simulink model "massbalancer"  (R2024a)
settings: Solver=VariableStepAuto  StartTime=0.0  StopTime=inf  RelTol=1e-3
libraries: matrix_library x36, sharedutil x2, sharedtransform x2, dspinverses x1, aerolibutil x1
(part 1 of 3)
settings Model: Creator=robertbergbaum  LastModifiedBy=robertbergbaum

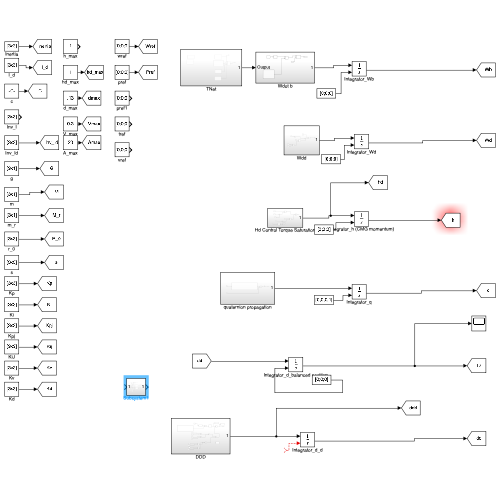
[thumbnail: Simulink's stored preview of the top-level diagram]
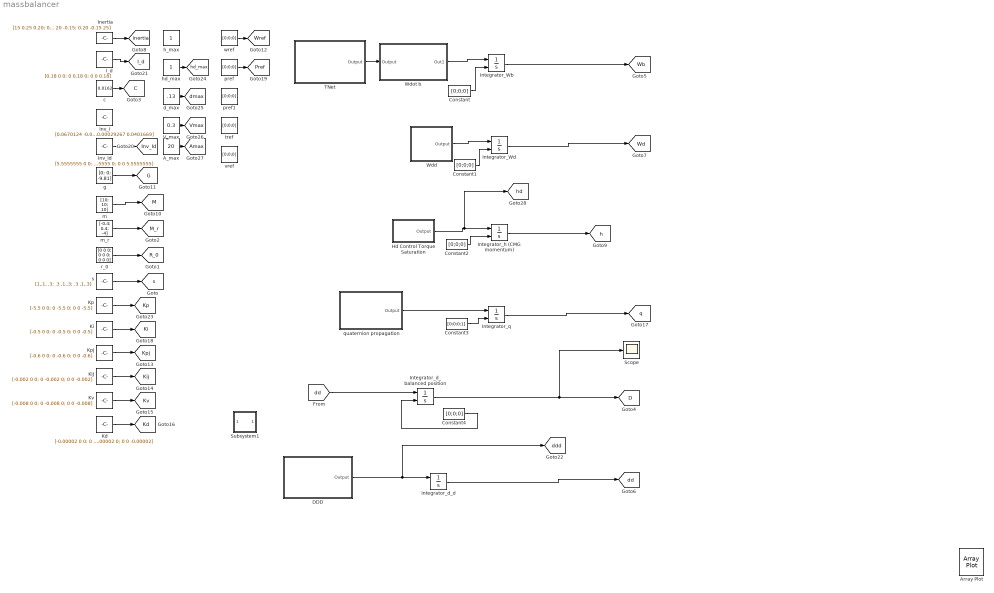
== system massbalancer ==
  A_max : Constant  Value=20
  Constant{,1..2,4} (4 alike) : Constant  Value=[0;0;0]  VectorParams1D=off
  Constant3 : Constant  Value=[0;0;0;1]  VectorParams1D=off
  DDD : Subsystem
  Hd Control Torque Saturation : Subsystem
  I_d : Constant  Value=[0.18 0 0; 0 0.18 0; 0 0 0.18]
  Inertia : Constant  Value=[15 0.25 0.20; 0.25 20 -0.15; 0.20 -0.15 25]  VectorParams1D=off
  Integrator_Wb : Integrator  InitialConditionSource=external  InitialCondition=[0;0;0]
  Integrator_Wd : Integrator  InitialConditionSource=external  InitialCondition=[0;0;0]
  Integrator_d_balanced position : Integrator  InitialConditionSource=external  InitialCondition=[0;0;0]
  Integrator_d_d : Integrator  InitialConditionSource=external  InitialCondition=[0;0;0]
  Integrator_h (CMG momentum) : Integrator  InitialConditionSource=external  InitialCondition=[0;0;0]
  Integrator_q : Integrator  InitialConditionSource=external  InitialCondition=[0;0;0;1]
  Inv_I : Constant  Value=[0.0670124 -0.0008106 -0.00051308; -0.0008106 0.0500357 0.00029267; -0.00051308 0.00029267 0.0401669]
  Inv_Id : Constant  Value=[5.5555555 0 0; 0 5.5555555 0; 0 0 5.5555555]
  Kd : Constant  Value=[-0.00002 0 0; 0 -0.00002 0; 0 0 -0.00002]
  Ki : Constant  Value=[-0.5 0 0; 0 -0.5 0; 0 0 -0.5]
  KiJ : Constant  Value=[-0.002 0 0; 0 -0.002 0; 0 0 -0.002]
  Kp : Constant  Value=[-5.5 0 0; 0 -5.5 0; 0 0 -5.5]
  Kpj : Constant  Value=[-0.6 0 0; 0 -0.6 0; 0 0 -0.6]
  Kv : Constant  Value=[-0.008 0 0; 0 -0.008 0; 0 0 -0.008]
  Scope : Scope
  Subsystem1 : Subsystem
  TNet : Subsystem
  V_max : Constant  Value=0.3
  Wdd : Subsystem
  Wdot b : Subsystem
  c : Constant  Value=0.0162  VectorParams1D=off
  d_max : Constant  Value=.13
  g : Constant  Value=[0; 0; -9.81]  VectorParams1D=off
  h_max : Constant
  hd_max : Constant
  m : Constant  Value=[10; 10; 10]  VectorParams1D=off
  m_r : Constant  Value=[-0.4; 0.4; -4]  VectorParams1D=off
  pref : Constant  Value=[0;0;0]  VectorParams1D=off
  pref1 : Constant  Value=[0;0;0]
  quaternion propagation : Subsystem
  r_0 : Constant  Value=[0 0 0; 0 0 0; 0 0 0]
  s : Constant  Value=[1,.1, .3; .3 ,1,.3; .3 ,1,.3]  VectorParams1D=off
  tref : Constant  Value=[0;0;0]
  vref : Constant  Value=[0;0;0]
  wref : Constant  Value=[0;0;0]  VectorParams1D=off
  Array Plot : ArrayPlot  IOType=viewer  IsFloating=on  WindowPosition=[447.000000,282.000000,800.000000,500.000000,]  ScopeFrameLocation=window  YLimits=[-4.3585 5.1367]  DefaultConfigurationName=dsp.scopes.ArrayPlotBlockSpecification
  tag scope: Amax=global, C=global, D=global, G=global, I_d=global, Inv_Id=global, Kd=global, Ki=global, Kij=global, Kp=global, Kpj=global, Kv=global, M=global, M_r=global, Pref=global, R_0=global, Vmax=global, Wb=global, Wd=global, Wref=global, dd=global, ddd=global, dmax=global, h=global, hd=global, hd_max=global, inertia=global, q=global, s=global
  wires:
  Integrator_Wb/1 -> [Wb]
  Kp/1 -> [Kp]
  Integrator_q/1 -> [q]
  Integrator_d_d/1 -> [dd]
  KiJ/1 -> [Kij]
  TNet/1(Output) -> Wdot b/1(Output)
  Ki/1 -> [Ki]
  s/1 -> [s]
  Constant2/1 -> Integrator_h (CMG momentum)/2
  r_0/1 -> [R_0]
  A_max/1 -> [Amax]
  Constant4/1 -> Integrator_d_balanced position/2
  I_d/1 -> [I_d]
  wref/1 -> [Wref]
  Inv_Id/1 -> [Inv_Id]
  [dd] -> Integrator_d_balanced position/1
  Wdot b/1(Out1) -> Integrator_Wb/1
  Integrator_d_balanced position/1 -> Scope/1, [D]
  DDD/1(Output) -> [ddd], Integrator_d_d/1
  Kd/1 -> [Kd]
  m/1 -> [M]
  pref/1 -> [Pref]
  Kpj/1 -> [Kpj]
  Kv/1 -> [Kv]
  Constant/1 -> Integrator_Wb/2
  Inertia/1 -> [inertia]
  c/1 -> [C]
  ? -> Integrator_d_d/2
  m_r/1 -> [M_r]
  Integrator_Wd/1 -> [Wd]
  Constant1/1 -> Integrator_Wd/2
  Wdd/1(Output) -> Integrator_Wd/1
  quaternion propagation/1(Output) -> Integrator_q/1
  g/1 -> [G]
  Hd Control Torque Saturation/1(Output) -> [hd], Integrator_h (CMG momentum)/1
  Integrator_h (CMG momentum)/1 -> [h]
  hd_max/1 -> [hd_max]
  Constant3/1 -> Integrator_q/2
  V_max/1 -> [Vmax]
  d_max/1 -> [dmax]

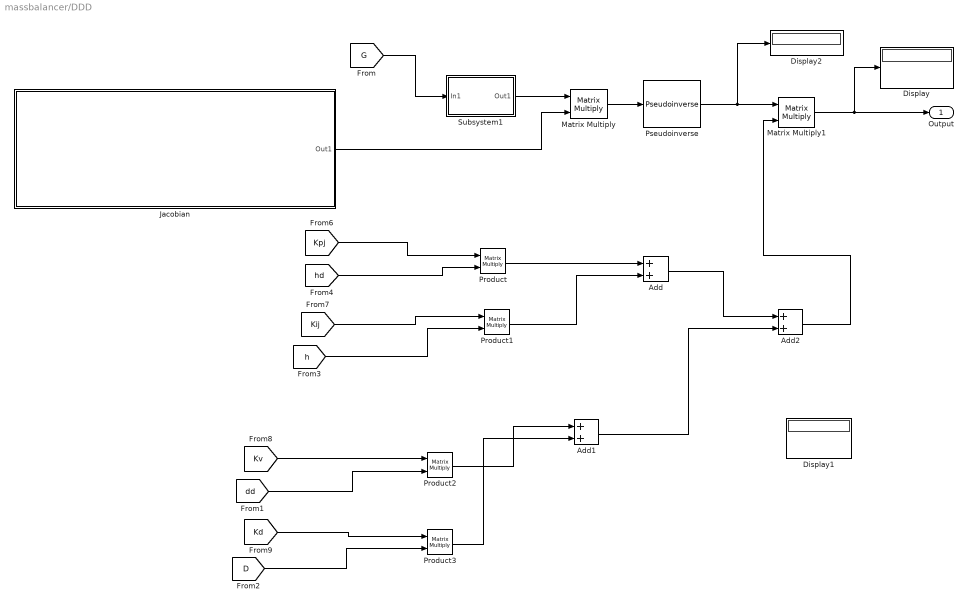
== system massbalancer/DDD ==
  Add : Sum
  Add1 : Sum
  Add2 : Sum
  Display : Display
  Display1 : Display
  Display2 : Display
  Jacobian : Subsystem
  Matrix Multiply : Product  Multiplication=Matrix(*)
  Matrix Multiply1 : Product  Multiplication=Matrix(*)
  Product{,1..3} (4 alike) : Product  Multiplication=Matrix(*)
  Pseudoinverse : dspinverses/Pseudoinverse  wanterr=off  SimulateUsing=Interpreted execution
  Subsystem1 : Subsystem
  Output : Outport
  wires:
  [Kij] -> Product1/1
  Add2/1 -> Matrix Multiply1/2
  Matrix Multiply/1 -> Pseudoinverse/1
  [Kpj] -> Product/1
  [h] -> Product1/2
  [G] -> Subsystem1/1(In1)
  [Kd] -> Product3/1
  [Kv] -> Product2/1
  [dd] -> Product2/2
  Subsystem1/1(Out1) -> Matrix Multiply/1
  Pseudoinverse/1 -> Display2/1, Matrix Multiply1/1
  Jacobian/1(Out1) -> Matrix Multiply/2
  Matrix Multiply1/1 -> Display/1, Output/1
  [D] -> Product3/2
  [hd] -> Product/2
  Product1/1 -> Add/2
  Product/1 -> Add/1
  Product2/1 -> Add1/1
  Product3/1 -> Add1/2
  Add/1 -> Add2/1
  Add1/1 -> Add2/2

== system massbalancer/Hd Control Torque Saturation ==
  Add : Sum
  Gain : Gain  Gain=2
  Matrix Multiply : Product  Multiplication=Matrix(*)
  Matrix Multiply1 : Product  Multiplication=Matrix(*)
  Selector : Selector  InputPortWidth=4  IndexOptions=Index vector (dialog)  Indices=[1 2 3]  OutputSizes=1
  Sum : Sum  Inputs=|+-
  Sum1 : Sum  Inputs=|+-
  Output : Outport
  wires:
  [q] -> Selector/1
  Selector/1 -> Gain/1
  Gain/1 -> Sum/2
  [Pref] -> Sum/1
  [Ki] -> Matrix Multiply/1
  Sum/1 -> Matrix Multiply/2
  [Wref] -> Sum1/1
  [Wb] -> Sum1/2
  [Kp] -> Matrix Multiply1/1
  Sum1/1 -> Matrix Multiply1/2
  Matrix Multiply1/1 -> Add/1
  Matrix Multiply/1 -> Add/2
  Add/1 -> Output/1

== system massbalancer/Subsystem1 ==
  In1 : Inport
  Demux : Demux  Outputs=3
  Demux1 : Demux  Outputs=3
  Demux4 : Demux  Outputs=3
  Mux : Mux  Inputs=3
  Subsystem1 : Subsystem
  Subsystem2 : Subsystem
  Subsystem3 : Subsystem
  Out1 : Outport
  wires:
  Demux/3 -> Subsystem3/6(ddd)
  Demux/2 -> Subsystem1/6(ddd)
  Demux/1 -> Subsystem2/5(ddd)
  Subsystem2/1(Out1) -> Mux/1
  Subsystem1/1(Out1) -> Mux/2
  Mux/1 -> Out1/1
  In1/1 -> Demux/1
  Subsystem3/1(Out1) -> Mux/3
  [D] -> Demux1/1
  Demux1/1 -> Subsystem2/1(d)
  [dd] -> Demux4/1
  Demux4/1 -> Subsystem2/3(dd)
  Demux1/2 -> Subsystem1/1(d)
  Demux4/2 -> Subsystem1/3(dd)
  [Amax] -> Subsystem2/6(amax), Subsystem1/5(amax), Subsystem3/5(amax)
  [Vmax] -> Subsystem3/4(vmax), Subsystem1/4(vmax), Subsystem2/4(vmax)
  Demux4/3 -> Subsystem3/3(dd)
  [dmax] -> Subsystem2/2(dmax), Subsystem3/2(dmax), Subsystem1/2(dmax)
  Demux1/3 -> Subsystem3/1(d)

== system massbalancer/TNet ==
  Add : Sum  Inputs=++--
  Hd Control Torque Saturation : Subsystem
  Subsystem : Subsystem
  Subsystem1 : Subsystem
  TBalances : Subsystem
  "Tbalances Init T Gravity " : Subsystem
  Tdamp : Subsystem
  Output : Outport
  tag scope: Tdamp=global
  wires:
  Tdamp/1(Outport) -> Add/1, [Tdamp]
  Subsystem/1(Out1) -> Add/3
  Hd Control Torque Saturation/1(Output) -> Add/4
  Add/1 -> Output/1
  Subsystem1/1(Output) -> Add/2

== system massbalancer/Wdd ==
  Cross Product : matrix_library/Cross Product
  Gain : Gain  Gain=-1
  Matrix Multiply : Product  Multiplication=Matrix(*)
  Matrix Multiply1 : Product  Multiplication=Matrix(*)
  Sum : Sum  Inputs=|+-
  Output : Outport
  wires:
  [Wb] -> Cross Product/1
  [Wd] -> Matrix Multiply/2
  [I_d] -> Matrix Multiply/1
  Matrix Multiply/1 -> Cross Product/2
  [Tdamp] -> Gain/1
  Gain/1 -> Sum/1
  Cross Product/1 -> Sum/2
  Sum/1 -> Matrix Multiply1/2
  [Inv_Id] -> Matrix Multiply1/1
  Matrix Multiply1/1 -> Output/1

== system massbalancer/Wdot b ==
  Output : Inport
  I_r : Subsystem
  Invert 3x3 Matrix : aerolibutil/Invert  3x3 Matrix
  Matrix Multiply : Product  Multiplication=Matrix(*)
  Subtract : Sum  Inputs=+-
  Out1 : Outport
  wires:
  Matrix Multiply/1 -> Out1/1
  I_r/1(Out1) -> Subtract/2
  Subtract/1 -> Matrix Multiply/1
  Output/1 -> Matrix Multiply/2
  [inertia] -> Invert 3x3 Matrix/1
  Invert 3x3 Matrix/1 -> Subtract/1

== system massbalancer/quaternion propagation ==
  Matrix Multiply : Product  Multiplication=Matrix(*)
  Multiply : Gain  Gain=0.5
  Omega Wb : Subsystem
  Output : Outport
  wires:
  [Wb] -> Omega Wb/1(In1)
  Multiply/1 -> Output/1
  Omega Wb/1(Output) -> Matrix Multiply/1
  Matrix Multiply/1 -> Multiply/1
  [q] -> Matrix Multiply/2

== system massbalancer/DDD/Jacobian ==
  Gain : Gain  Gain=-1
  Matrix Concatenate : Concatenate  NumInputs=3  Mode=Multidimensional array  ConcatenateDimension=2
  Product : Product
  Product1 : Product
  Product2 : Product
  Selector : Selector  InputPortWidth=3  IndexOptions=Index vector (dialog)  Indices=[1]  OutputSizes=1
  Selector1 : Selector  InputPortWidth=3  IndexOptions=Index vector (dialog)  Indices=[2]  OutputSizes=1
  Selector2 : Selector  InputPortWidth=3  IndexOptions=Index vector (dialog)  Indices=[3]  OutputSizes=1
  Subsystem1 : Subsystem
  Out1 : Outport
  wires:
  Product1/1 -> Matrix Concatenate/2
  Subsystem1/2(Out2) -> Product1/1
  Subsystem1/1(Out1) -> Product/1
  Product2/1 -> Matrix Concatenate/3
  Selector2/1 -> Product2/2
  Selector/1 -> Product/2
  Matrix Concatenate/1 -> Gain/1
  Selector1/1 -> Product1/2
  [M] -> Selector/1, Selector2/1, Selector1/1
  Gain/1 -> Out1/1
  Product/1 -> Matrix Concatenate/1
  Subsystem1/3(Out3) -> Product2/1
  [s] -> Subsystem1/1(R_0)

== system massbalancer/DDD/Subsystem1 ==
  In1 : Inport
  Constant : Constant  Value=0  VectorParams1D=off
  Constant1 : Constant  Value=0  VectorParams1D=off
  Constant2 : Constant  Value=0  VectorParams1D=off
  Demux : Demux  Outputs=3
  Gain : Gain  Gain=-1
  Gain1 : Gain  Gain=-1
  Gain2 : Gain  Gain=-1
  Matrix Concatenate : Concatenate  NumInputs=3  Mode=Multidimensional array  ConcatenateDimension=2
  Mux : Mux  Inputs=3
  Mux1 : Mux  Inputs=3
  Mux2 : Mux  Inputs=3
  Out1 : Outport
  wires:
  Matrix Concatenate/1 -> Out1/1
  Constant2/1 -> Mux2/3
  Constant1/1 -> Mux1/2
  Demux/1 -> Gain1/1, Mux2/2
  Mux2/1 -> Matrix Concatenate/3
  Demux/3 -> Gain/1, Mux1/1
  Gain/1 -> Mux/2
  In1/1 -> Demux/1
  Demux/2 -> Gain2/1, Mux/3
  Mux/1 -> Matrix Concatenate/1
  Gain1/1 -> Mux1/3
  Gain2/1 -> Mux2/1
  Constant/1 -> Mux/1
  Mux1/1 -> Matrix Concatenate/2

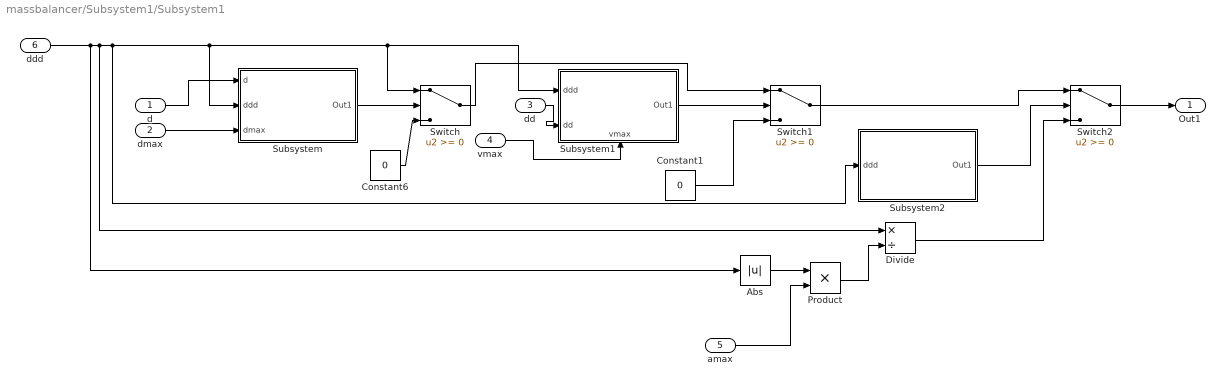
== system massbalancer/Subsystem1/Subsystem1 ==
  d : Inport
  dmax : Inport  Port=2
  dd : Inport  Port=3
  vmax : Inport  Port=4
  amax : Inport  Port=5
  ddd : Inport  Port=6
  Abs : Abs  SaturateOnIntegerOverflow=off
  Constant1 : Constant  Value=0  VectorParams1D=off
  Constant6 : Constant  Value=0  VectorParams1D=off
  Divide : Product  Inputs=*/
  Product : Product
  Subsystem : Subsystem
  Subsystem1 : Subsystem
      settings: PortSchema="{\"entries\":[{\"content\":{\"sides\":[{\"content\":{\"connectorIds\":[\"In1\",\"In2\"]},\"type\":\"ConnectorPlacement.EquallySpacedRectSide\",\"uuid\":\"8ae5d5fe-f648-4880-a31b-82c697ea1f6b\"},{\"content\":{\"connectorIds\":[\"Out1\"],\"side\":\"RIGHT\"},\"type\":\"ConnectorPlacement.EquallySpacedRectSide\",\"uuid\":\"93459a1a-512a-419a-be8d-aafe7ca608a5\"},{\"content\":{\"side\":\"TOP\"},\"type\":\"ConnectorPlacement.EquallySpacedRectSide\",\"uuid\":\"819310a9-1bbe-4933-988e-a24734f33f30\"},{\"content\":{\"connectorIds\":[\"In3\"],\"side\":\"BOTTOM\"},\"type\":\"ConnectorPlacement.EquallySpacedRectSide\",\"uuid\":\"b19b6ff1-25c5-41e7-8899-8dec42881787\"}]},\"type\":\"ConnectorPlacement.EquallySpacedConnector\",\"uuid\":\"36ccd371-697e-4cae-b4c0-046b64d9372c\"}],\"packageUris\":[\"http://schema.mathworks.com/mf0/Connector/R2020b\"],\"version\":\"1.0\"}"
  Subsystem2 : Subsystem
  Switch : Switch  SaturateOnIntegerOverflow=off  InputSameDT=off
  Switch1 : Switch  SaturateOnIntegerOverflow=off  InputSameDT=off
  Switch2 : Switch  SaturateOnIntegerOverflow=off  InputSameDT=off
  Out1 : Outport
  wires:
  vmax/1 -> Subsystem1/3(vmax)
  dd/1 -> Subsystem1/2(dd)
  dmax/1 -> Subsystem/3(dmax)
  d/1 -> Subsystem/1(d)
  Switch1/1 -> Switch2/1
  Switch/1 -> Switch1/1
  Constant6/1 -> Switch/3
  Product/1 -> Divide/2
  Switch2/1 -> Out1/1
  Divide/1 -> Switch2/3
  ddd/1 -> Switch/1, Subsystem1/1(ddd), Subsystem/2(ddd), Subsystem2/1(ddd), Divide/1, Abs/1
  Subsystem/1(Out1) -> Switch/2
  Subsystem2/1(Out1) -> Switch2/2
  amax/1 -> Product/2
  Subsystem1/1(Out1) -> Switch1/2
  Constant1/1 -> Switch1/3
  Abs/1 -> Product/1

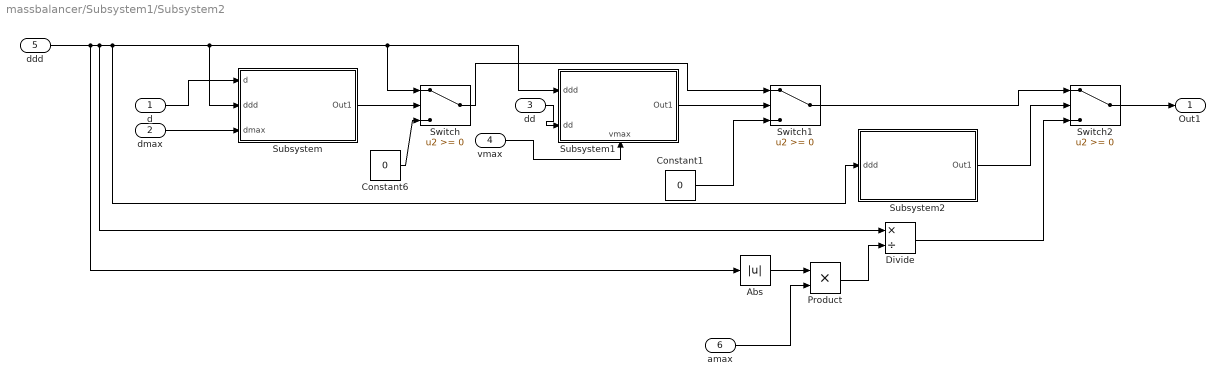
== system massbalancer/Subsystem1/Subsystem2 ==
  d : Inport
  dmax : Inport  Port=2
  dd : Inport  Port=3
  vmax : Inport  Port=4
  ddd : Inport  Port=5
  amax : Inport  Port=6
  Abs : Abs  SaturateOnIntegerOverflow=off
  Constant1 : Constant  Value=0  VectorParams1D=off
  Constant6 : Constant  Value=0  VectorParams1D=off
  Divide : Product  Inputs=*/
  Product : Product
  Subsystem : Subsystem
  Subsystem1 : Subsystem
      settings: PortSchema="{\"entries\":[{\"content\":{\"sides\":[{\"content\":{\"connectorIds\":[\"In1\",\"In2\"]},\"type\":\"ConnectorPlacement.EquallySpacedRectSide\",\"uuid\":\"8ae5d5fe-f648-4880-a31b-82c697ea1f6b\"},{\"content\":{\"connectorIds\":[\"Out1\"],\"side\":\"RIGHT\"},\"type\":\"ConnectorPlacement.EquallySpacedRectSide\",\"uuid\":\"93459a1a-512a-419a-be8d-aafe7ca608a5\"},{\"content\":{\"side\":\"TOP\"},\"type\":\"ConnectorPlacement.EquallySpacedRectSide\",\"uuid\":\"819310a9-1bbe-4933-988e-a24734f33f30\"},{\"content\":{\"connectorIds\":[\"In3\"],\"side\":\"BOTTOM\"},\"type\":\"ConnectorPlacement.EquallySpacedRectSide\",\"uuid\":\"b19b6ff1-25c5-41e7-8899-8dec42881787\"}]},\"type\":\"ConnectorPlacement.EquallySpacedConnector\",\"uuid\":\"36ccd371-697e-4cae-b4c0-046b64d9372c\"}],\"packageUris\":[\"http://schema.mathworks.com/mf0/Connector/R2020b\"],\"version\":\"1.0\"}"
  Subsystem2 : Subsystem
  Switch : Switch  SaturateOnIntegerOverflow=off  InputSameDT=off
  Switch1 : Switch  SaturateOnIntegerOverflow=off  InputSameDT=off
  Switch2 : Switch  SaturateOnIntegerOverflow=off  InputSameDT=off
  Out1 : Outport
  wires:
  Abs/1 -> Product/1
  Constant1/1 -> Switch1/3
  Subsystem1/1(Out1) -> Switch1/2
  amax/1 -> Product/2
  Subsystem2/1(Out1) -> Switch2/2
  Subsystem/1(Out1) -> Switch/2
  ddd/1 -> Abs/1, Divide/1, Subsystem2/1(ddd), Subsystem/2(ddd), Subsystem1/1(ddd), Switch/1
  Divide/1 -> Switch2/3
  Switch2/1 -> Out1/1
  Product/1 -> Divide/2
  Constant6/1 -> Switch/3
  Switch/1 -> Switch1/1
  Switch1/1 -> Switch2/1
  d/1 -> Subsystem/1(d)
  dmax/1 -> Subsystem/3(dmax)
  dd/1 -> Subsystem1/2(dd)
  vmax/1 -> Subsystem1/3(vmax)

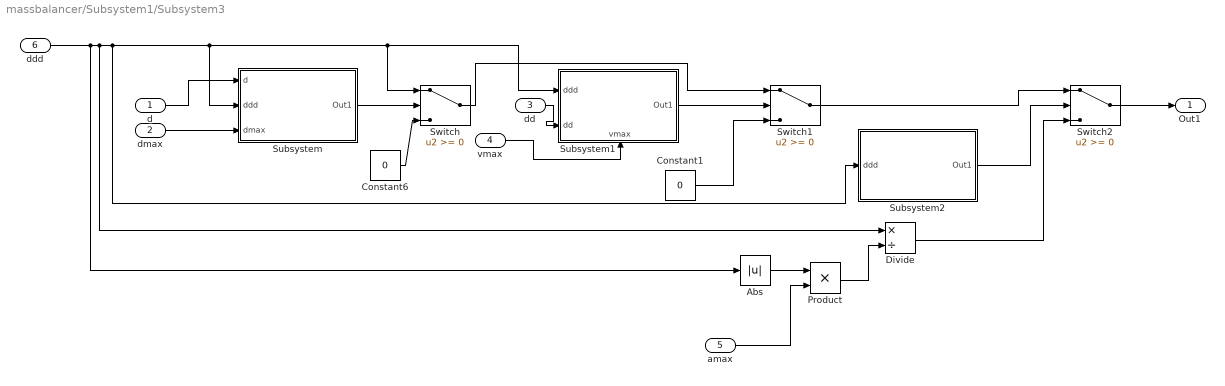
== system massbalancer/Subsystem1/Subsystem3 ==
  d : Inport
  dmax : Inport  Port=2
  dd : Inport  Port=3
  vmax : Inport  Port=4
  amax : Inport  Port=5
  ddd : Inport  Port=6
  Abs : Abs  SaturateOnIntegerOverflow=off
  Constant1 : Constant  Value=0  VectorParams1D=off
  Constant6 : Constant  Value=0  VectorParams1D=off
  Divide : Product  Inputs=*/
  Product : Product
  Subsystem : Subsystem
  Subsystem1 : Subsystem
      settings: PortSchema="{\"entries\":[{\"content\":{\"sides\":[{\"content\":{\"connectorIds\":[\"In1\",\"In2\"]},\"type\":\"ConnectorPlacement.EquallySpacedRectSide\",\"uuid\":\"8ae5d5fe-f648-4880-a31b-82c697ea1f6b\"},{\"content\":{\"connectorIds\":[\"Out1\"],\"side\":\"RIGHT\"},\"type\":\"ConnectorPlacement.EquallySpacedRectSide\",\"uuid\":\"93459a1a-512a-419a-be8d-aafe7ca608a5\"},{\"content\":{\"side\":\"TOP\"},\"type\":\"ConnectorPlacement.EquallySpacedRectSide\",\"uuid\":\"819310a9-1bbe-4933-988e-a24734f33f30\"},{\"content\":{\"connectorIds\":[\"In3\"],\"side\":\"BOTTOM\"},\"type\":\"ConnectorPlacement.EquallySpacedRectSide\",\"uuid\":\"b19b6ff1-25c5-41e7-8899-8dec42881787\"}]},\"type\":\"ConnectorPlacement.EquallySpacedConnector\",\"uuid\":\"36ccd371-697e-4cae-b4c0-046b64d9372c\"}],\"packageUris\":[\"http://schema.mathworks.com/mf0/Connector/R2020b\"],\"version\":\"1.0\"}"
  Subsystem2 : Subsystem
  Switch : Switch  SaturateOnIntegerOverflow=off  InputSameDT=off
  Switch1 : Switch  SaturateOnIntegerOverflow=off  InputSameDT=off
  Switch2 : Switch  SaturateOnIntegerOverflow=off  InputSameDT=off
  Out1 : Outport
  wires:
  Abs/1 -> Product/1
  Constant1/1 -> Switch1/3
  Subsystem1/1(Out1) -> Switch1/2
  amax/1 -> Product/2
  Subsystem2/1(Out1) -> Switch2/2
  Subsystem/1(Out1) -> Switch/2
  ddd/1 -> Abs/1, Divide/1, Subsystem2/1(ddd), Subsystem/2(ddd), Subsystem1/1(ddd), Switch/1
  Divide/1 -> Switch2/3
  Switch2/1 -> Out1/1
  Product/1 -> Divide/2
  Constant6/1 -> Switch/3
  Switch/1 -> Switch1/1
  Switch1/1 -> Switch2/1
  d/1 -> Subsystem/1(d)
  dmax/1 -> Subsystem/3(dmax)
  dd/1 -> Subsystem1/2(dd)
  vmax/1 -> Subsystem1/3(vmax)

== system massbalancer/TNet/Hd Control Torque Saturation ==
  Add : Sum
  Gain : Gain  Gain=2
  Matrix Multiply : Product  Multiplication=Matrix(*)
  Matrix Multiply1 : Product  Multiplication=Matrix(*)
  Selector : Selector  InputPortWidth=4  IndexOptions=Index vector (dialog)  Indices=[1 2 3]  OutputSizes=1
  Sum : Sum  Inputs=|+-
  Sum1 : Sum  Inputs=|+-
  Output : Outport
  wires:
  [q] -> Selector/1
  Selector/1 -> Gain/1
  Gain/1 -> Sum/2
  [Pref] -> Sum/1
  [Ki] -> Matrix Multiply/1
  Sum/1 -> Matrix Multiply/2
  [Wref] -> Sum1/1
  [Wb] -> Sum1/2
  [Kp] -> Matrix Multiply1/1
  Sum1/1 -> Matrix Multiply1/2
  Matrix Multiply1/1 -> Add/1
  Matrix Multiply/1 -> Add/2
  Add/1 -> Output/1

== system massbalancer/TNet/Subsystem ==
  Cross Product : matrix_library/Cross Product
  Product : Product  Multiplication=Matrix(*)
  Sum : Sum  Inputs=|++
  Out1 : Outport
  wires:
  Product/1 -> Sum/1
  [h] -> Sum/2
  Cross Product/1 -> Out1/1
  [inertia] -> Product/1
  Sum/1 -> Cross Product/2
  [Wb] -> Cross Product/1
  [Wb] -> Product/2

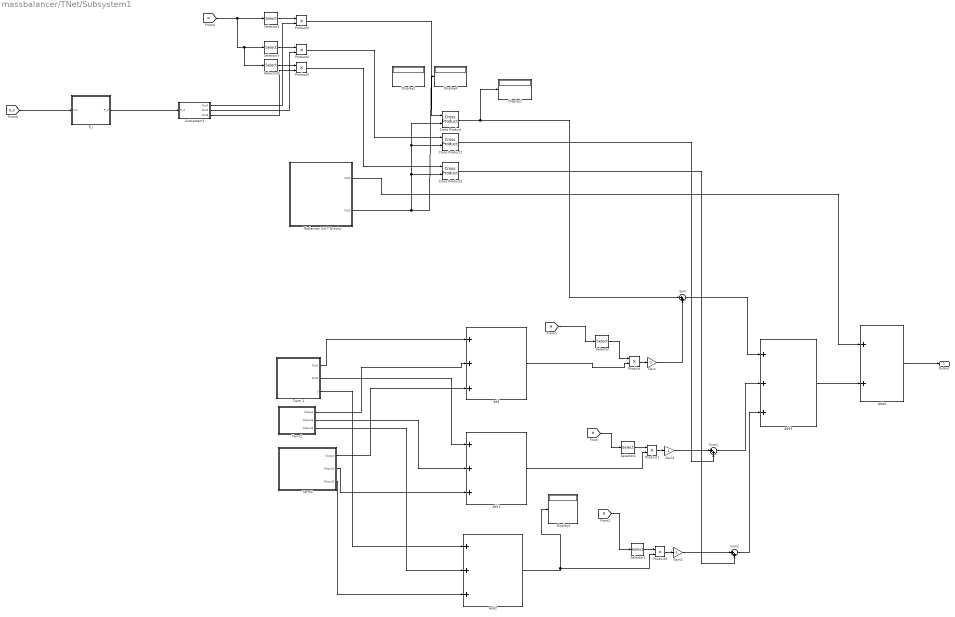
== system massbalancer/TNet/Subsystem1 ==
  Add{,1..3} (4 alike) : Sum  Inputs=+++
  Add4 : Sum
  Cross Product : matrix_library/Cross Product
  Cross Product1 : matrix_library/Cross Product
  Cross Product2 : matrix_library/Cross Product
  Display{1..4} (4 alike) : Display
  Gain : Gain  Gain=-1
  Gain1 : Gain  Gain=-1
  Gain2 : Gain  Gain=-1
  Product{,1..5} (6 alike) : Product
  R_I : Subsystem
  Selector : Selector  InputPortWidth=3  IndexOptions=Index vector (dialog)  Indices=[1]  OutputSizes=1
  Selector1 : Selector  InputPortWidth=3  IndexOptions=Index vector (dialog)  Indices=[2]  OutputSizes=1
  Selector2 : Selector  InputPortWidth=3  IndexOptions=Index vector (dialog)  Indices=[3]  OutputSizes=1
  Selector3 : Selector  InputPortWidth=3  IndexOptions=Index vector (dialog)  Indices=[2]  OutputSizes=1
  Selector4 : Selector  InputPortWidth=3  IndexOptions=Index vector (dialog)  Indices=[1]  OutputSizes=1
  Selector5 : Selector  InputPortWidth=3  IndexOptions=Index vector (dialog)  Indices=[3]  OutputSizes=1
  Subsystem3 : Subsystem
  Sum : Sum  Inputs=|++
  Sum1 : Sum  Inputs=|++
  Sum2 : Sum  Inputs=|++
  "Tbalances Init T Gravity " : Subsystem
  Term 1 : Subsystem
  Term2 : Subsystem
  Term3 : Subsystem
  Output : Outport
  wires:
  [M] -> Selector2/1
  Product2/1 -> Gain2/1
  Term 1/3(y) -> Add2/1
  Add1/1 -> Product1/2
  Sum1/1 -> Add3/2
  Add3/1 -> Add4/2
  Subsystem3/2(Out2) -> Product4/2
  Sum2/1 -> Add3/3
  "Tbalances Init T Gravity "/1(Out1) -> Add4/1
  Term3/2(Output1) -> Add1/3
  Subsystem3/3(Out3) -> Product5/2
  Cross Product/1 -> Display1/1, Sum/1
  Product4/1 -> Cross Product1/1
  Add4/1 -> Output/1
  Gain1/1 -> Sum1/1
  Cross Product2/1 -> Sum2/2
  [M] -> Selector1/1
  R_I/1(R_0) -> Subsystem3/1(R_0)
  Term2/1(Output) -> Add/2
  Term2/3(Output2) -> Add2/2
  Product5/1 -> Cross Product2/1
  Cross Product1/1 -> Sum1/2
  [M] -> Selector5/1, Selector3/1, Selector4/1
  Selector2/1 -> Product2/1
  Term2/2(Output1) -> Add1/2
  Term 1/1(Out1) -> Add/1
  Term3/1(Output) -> Add/3
  [R_0] -> R_I/1(In1)
  Selector4/1 -> Product3/1
  [M] -> Selector/1
  Product/1 -> Gain/1
  Term3/3(Output2) -> Add2/3
  "Tbalances Init T Gravity "/2(Out2) -> Display4/1, Cross Product2/2, Cross Product1/2, Cross Product/2
  Subsystem3/1(Out1) -> Product3/2
  Gain2/1 -> Sum2/1
  Selector/1 -> Product/1
  Add/1 -> Product/2
  Add2/1 -> Product2/2, Display3/1
  Term 1/2(Out2) -> Add1/1
  Selector3/1 -> Product4/1
  Product1/1 -> Gain1/1
  Product3/1 -> Cross Product/1
  Selector1/1 -> Product1/1
  Gain/1 -> Sum/2
  Selector5/1 -> Product5/1
  Sum/1 -> Add3/1

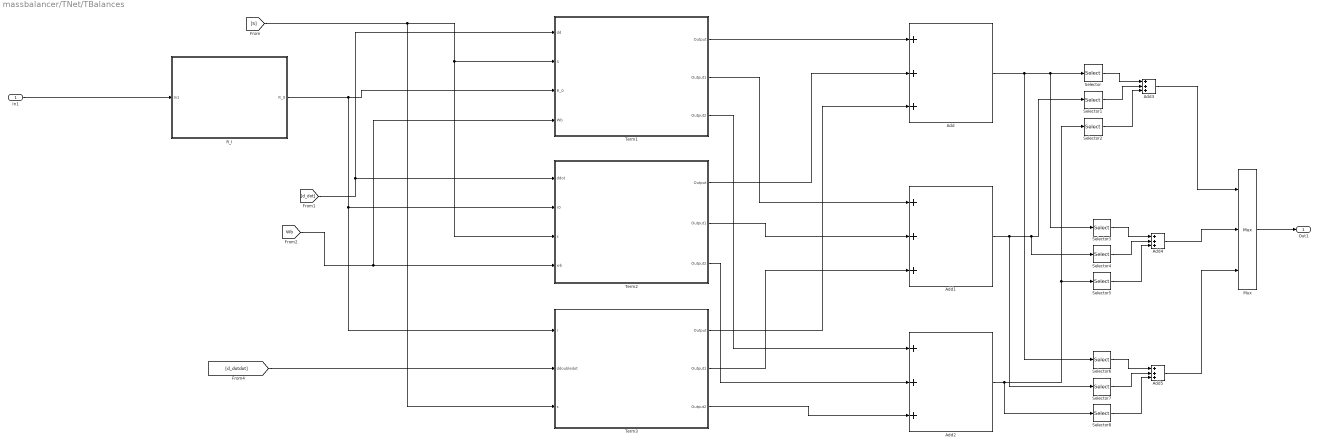
== system massbalancer/TNet/TBalances ==
  In1 : Inport
  Add{,1..5} (6 alike) : Sum  Inputs=+++
  Mux : Mux  Inputs=3
  R_I : Subsystem
  Selector : Selector  InputPortWidth=3  IndexOptions=Index vector (dialog)  Indices=[1 ]  OutputSizes=1
  Selector1 : Selector  InputPortWidth=3  IndexOptions=Index vector (dialog)  Indices=[1 ]  OutputSizes=1
  Selector2 : Selector  InputPortWidth=3  IndexOptions=Index vector (dialog)  Indices=[1 ]  OutputSizes=1
  Selector3 : Selector  InputPortWidth=3  IndexOptions=Index vector (dialog)  Indices=[2 ]  OutputSizes=1
  Selector4 : Selector  InputPortWidth=3  IndexOptions=Index vector (dialog)  Indices=[2]  OutputSizes=1
  Selector5 : Selector  InputPortWidth=3  IndexOptions=Index vector (dialog)  Indices=[2 ]  OutputSizes=1
  Selector6 : Selector  InputPortWidth=3  IndexOptions=Index vector (dialog)  Indices=[3 ]  OutputSizes=1
  Selector7 : Selector  InputPortWidth=3  IndexOptions=Index vector (dialog)  Indices=[3]  OutputSizes=1
  Selector8 : Selector  InputPortWidth=3  IndexOptions=Index vector (dialog)  Indices=[3 ]  OutputSizes=1
  Term1 : Subsystem
  Term2 : Subsystem
  Term3 : Subsystem
  Out1 : Outport
  wires:
  Add2/1 -> Selector8/1, Selector5/1, Selector2/1
  [d_dotdot] -> Term3/2(ddoubledot)
  Term1/3(Output2) -> Add2/1
  Add3/1 -> Mux/1
  Add4/1 -> Mux/2
  Selector7/1 -> Add5/2
  Term3/2(Output1) -> Add1/3
  [d_dot] -> Term2/1(ddot), Term1/1(dd)
  Term1/1(Output) -> Add/1
  Term2/1(Output) -> Add/2
  [S] -> Term3/3(s), Term2/3(s), Term1/2(S)
  Selector2/1 -> Add3/3
  Selector8/1 -> Add5/3
  Term3/1(Output) -> Add/3
  Selector/1 -> Add3/1
  Term2/2(Output1) -> Add1/2
  Add/1 -> Selector6/1, Selector3/1, Selector/1
  Selector3/1 -> Add4/1
  Add1/1 -> Selector7/1, Selector4/1, Selector1/1
  Selector1/1 -> Add3/2
  Selector4/1 -> Add4/2
  Selector6/1 -> Add5/1
  Term1/2(Output1) -> Add1/1
  Term3/3(Output2) -> Add2/3
  R_I/1(R_0) -> Term3/1(r), Term2/2(r0), Term1/3(R_0)
  [Wb] -> Term1/4(Wb), Term2/4(wb)
  Selector5/1 -> Add4/3
  Term2/3(Output2) -> Add2/2
  Add5/1 -> Mux/3
  In1/1 -> R_I/1(In1)
  Mux/1 -> Out1/1

== system massbalancer/TNet/Tbalances Init T Gravity  ==
  Fgravity : Subsystem
  Matrix Multiply : Product  Multiplication=Matrix(*)
  Subsystem : Subsystem
  Out1 : Outport
  wires:
  Subsystem/1(Output) -> Matrix Multiply/1
  Fgravity/1(Out1) -> Matrix Multiply/2
  Matrix Multiply/1 -> Out1/1

== system massbalancer/TNet/Tdamp ==
  Product : Product
  Subtract : Sum  Inputs=+-
  Outport : Outport
  wires:
  [Wb] -> Subtract/2
  [Wd] -> Subtract/1
  Subtract/1 -> Product/1
  [C] -> Product/2
  Product/1 -> Outport/1

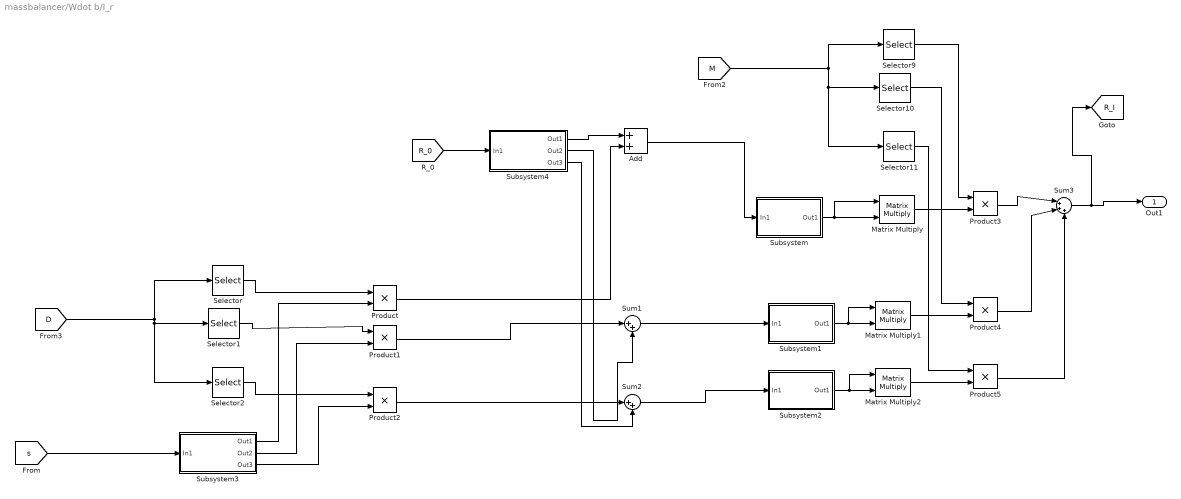
== system massbalancer/Wdot b/I_r ==
  Add : Sum
  Matrix Multiply : Product  Multiplication=Matrix(*)
  Matrix Multiply1 : Product  Multiplication=Matrix(*)
  Matrix Multiply2 : Product  Multiplication=Matrix(*)
  Product{,1..5} (6 alike) : Product
  Selector : Selector  InputPortWidth=3  IndexOptions=Index vector (dialog)  Indices=[1]  OutputSizes=1
  Selector1 : Selector  InputPortWidth=3  IndexOptions=Index vector (dialog)  Indices=[2]  OutputSizes=1
  Selector10 : Selector  InputPortWidth=3  IndexOptions=Index vector (dialog)  Indices=[2]  OutputSizes=1
  Selector11 : Selector  InputPortWidth=3  IndexOptions=Index vector (dialog)  Indices=[3]  OutputSizes=1
  Selector2 : Selector  InputPortWidth=3  IndexOptions=Index vector (dialog)  Indices=[3]  OutputSizes=1
  Selector9 : Selector  InputPortWidth=3  IndexOptions=Index vector (dialog)  Indices=[1]  OutputSizes=1
  Subsystem : Subsystem
  Subsystem1 : Subsystem
  Subsystem2 : Subsystem
  Subsystem3 : Subsystem
  Subsystem4 : Subsystem
  Sum1 : Sum  Inputs=|++
  Sum2 : Sum  Inputs=|++
  Sum3 : Sum  Inputs=|+++
  Out1 : Outport
  tag scope: R_I=global
  wires:
  Selector11/1 -> Product5/1
  Selector10/1 -> Product4/1
  Subsystem4/1(Out1) -> Add/1
  Subsystem/1(Out1) -> Matrix Multiply/1, Matrix Multiply/2
  Selector9/1 -> Product3/1
  Sum2/1 -> Subsystem2/1(In1)
  Matrix Multiply/1 -> Product3/2
  Matrix Multiply1/1 -> Product4/2
  Sum1/1 -> Subsystem1/1(In1)
  Product1/1 -> Sum1/1
  [M] -> Selector9/1, Selector11/1, Selector10/1
  Selector1/1 -> Product1/1
  Matrix Multiply2/1 -> Product5/2
  Add/1 -> Subsystem/1(In1)
  Selector/1 -> Product/1
  Product4/1 -> Sum3/2
  Subsystem3/2(Out2) -> Product1/2
  Product3/1 -> Sum3/1
  Selector2/1 -> Product2/1
  Subsystem4/2(Out2) -> Sum1/2
  [D] -> Selector/1, Selector1/1, Selector2/1
  Sum3/1 -> [R_I], Out1/1
  Product5/1 -> Sum3/3
  Subsystem4/3(Out3) -> Sum2/2
  Product/1 -> Add/2
  Subsystem3/1(Out1) -> Product/2
  [s] -> Subsystem3/1(In1)
  Subsystem3/3(Out3) -> Product2/2
  Subsystem2/1(Out1) -> Matrix Multiply2/1, Matrix Multiply2/2
  Product2/1 -> Sum2/1
  Subsystem1/1(Out1) -> Matrix Multiply1/1, Matrix Multiply1/2
  [R_0] -> Subsystem4/1(In1)

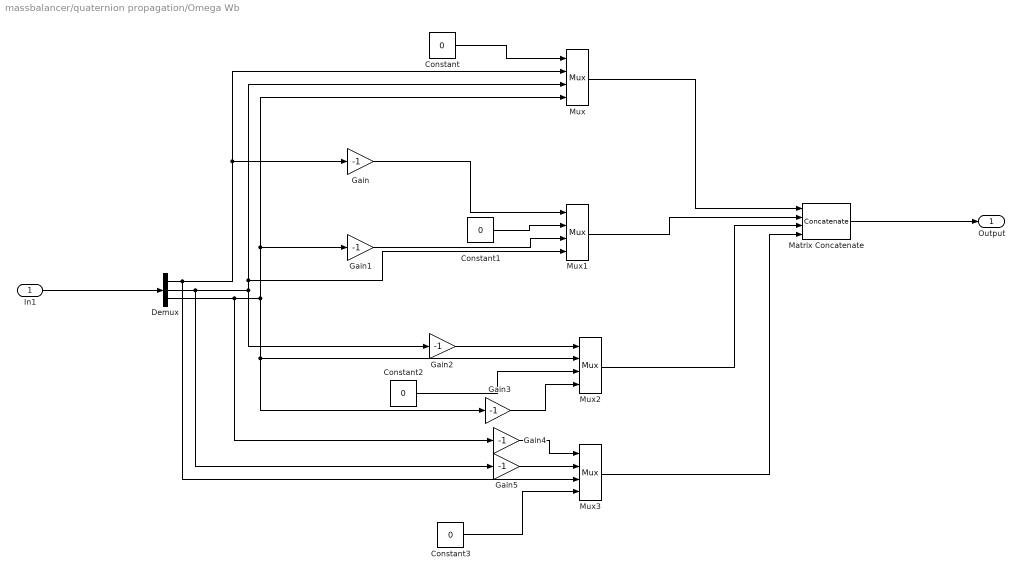
== system massbalancer/quaternion propagation/Omega Wb ==
  In1 : Inport
  Constant{,1..3} (4 alike) : Constant  Value=0  VectorParams1D=off
  Demux : Demux  Outputs=3
  Gain{,1..5} (6 alike) : Gain  Gain=-1
  Matrix Concatenate : Concatenate  NumInputs=4  Mode=Multidimensional array  ConcatenateDimension=2
  Mux{,1..3} (4 alike) : Mux
  Output : Outport
  wires:
  Constant/1 -> Mux/1
  In1/1 -> Demux/1
  Constant1/1 -> Mux1/2
  Gain1/1 -> Mux1/3
  Gain5/1 -> Mux3/2
  Gain/1 -> Mux1/1
  Mux2/1 -> Matrix Concatenate/3
  Demux/3 -> Gain4/1, Gain3/1, Mux2/2, Gain1/1, Mux/4
  Constant3/1 -> Mux3/4
  Constant2/1 -> Mux2/3
  Gain2/1 -> Mux2/1
  Mux3/1 -> Matrix Concatenate/4
  Gain4/1 -> Mux3/1
  Mux1/1 -> Matrix Concatenate/2
  Demux/1 -> Mux3/3, Gain/1, Mux/2
  Demux/2 -> Gain5/1, Mux/3, Mux1/4, Gain2/1
  Mux/1 -> Matrix Concatenate/1
  Gain3/1 -> Mux2/4
  Matrix Concatenate/1 -> Output/1

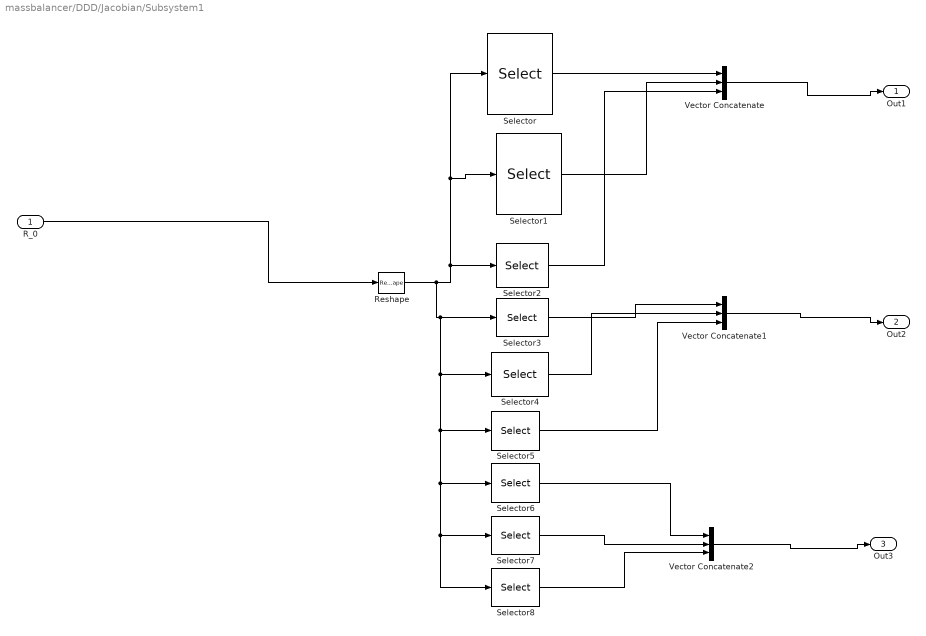
== system massbalancer/DDD/Jacobian/Subsystem1 ==
  R_0 : Inport
  Reshape : Reshape  OutputDimensionality=Column vector (2-D)  OutputDimensions=[1,3]
  Selector : Selector  InputPortWidth=9  IndexOptions=Index vector (dialog)  Indices=[1]  OutputSizes=1
  Selector1 : Selector  InputPortWidth=9  IndexOptions=Index vector (dialog)  Indices=[2]  OutputSizes=1
  Selector2 : Selector  InputPortWidth=9  IndexOptions=Index vector (dialog)  Indices=[3]  OutputSizes=1
  Selector3 : Selector  InputPortWidth=9  IndexOptions=Index vector (dialog)  Indices=[4]  OutputSizes=1
  Selector4 : Selector  InputPortWidth=9  IndexOptions=Index vector (dialog)  Indices=[5]  OutputSizes=1
  Selector5 : Selector  InputPortWidth=9  IndexOptions=Index vector (dialog)  Indices=[6]  OutputSizes=1
  Selector6 : Selector  InputPortWidth=9  IndexOptions=Index vector (dialog)  Indices=[7]  OutputSizes=1
  Selector7 : Selector  InputPortWidth=9  IndexOptions=Index vector (dialog)  Indices=[8]  OutputSizes=1
  Selector8 : Selector  InputPortWidth=9  IndexOptions=Index vector (dialog)  Indices=[9]  OutputSizes=1
  Vector Concatenate : Concatenate  NumInputs=3  Mode=Multidimensional array
  Vector Concatenate1 : Concatenate  NumInputs=3  Mode=Multidimensional array
  Vector Concatenate2 : Concatenate  NumInputs=3  Mode=Multidimensional array
  Out1 : Outport
  Out2 : Outport  Port=2
  Out3 : Outport  Port=3
  wires:
  Selector3/1 -> Vector Concatenate1/1
  Selector1/1 -> Vector Concatenate/2
  Vector Concatenate1/1 -> Out2/1
  Vector Concatenate2/1 -> Out3/1
  Selector7/1 -> Vector Concatenate2/2
  Selector5/1 -> Vector Concatenate1/3
  Selector/1 -> Vector Concatenate/1
  Reshape/1 -> Selector/1, Selector1/1, Selector2/1, Selector3/1, Selector4/1, Selector5/1, Selector6/1, Selector7/1, Selector8/1
  R_0/1 -> Reshape/1
  Selector6/1 -> Vector Concatenate2/1
  Selector4/1 -> Vector Concatenate1/2
  Selector8/1 -> Vector Concatenate2/3
  Vector Concatenate/1 -> Out1/1
  Selector2/1 -> Vector Concatenate/3

== system massbalancer/Subsystem1/Subsystem1/Subsystem ==
  d : Inport
  ddd : Inport  Port=2
  dmax : Inport  Port=3
  AND : Logic  IconShape=distinctive  AllPortsSameDT=off  OutDataTypeStr=boolean
  Abs : Abs  SaturateOnIntegerOverflow=off
  Constant : Constant  Value=0  VectorParams1D=off
  Constant1 : Constant  Value=0  VectorParams1D=off
  Enabled Subsystem : Subsystem  TreatAsAtomicUnit=on
  LessThanOrEqual : RelationalOperator  OutDataTypeStr=boolean  RndMeth=Simplest  InputSameDT=off
  LessThanOrEqual1 : RelationalOperator  OutDataTypeStr=boolean  RndMeth=Simplest  InputSameDT=off
  Product : Product
  Out1 : Outport
  wires:
  Abs/1 -> LessThanOrEqual/1
  d/1 -> Abs/1, Product/1
  Constant1/1 -> Enabled Subsystem/1(In1)
  LessThanOrEqual1/1 -> AND/2
  Constant/1 -> LessThanOrEqual1/2
  Product/1 -> LessThanOrEqual1/1
  ddd/1 -> Product/2
  dmax/1 -> LessThanOrEqual/2
  LessThanOrEqual/1 -> AND/1
  Enabled Subsystem/1(Out1) -> Out1/1
  AND/1 -> Enabled Subsystem/Enable

== system massbalancer/Subsystem1/Subsystem1/Subsystem1 ==
  ddd : Inport
  dd : Inport  Port=2
  vmax : Inport  Port=3
  AND : Logic  IconShape=distinctive  AllPortsSameDT=off  OutDataTypeStr=boolean
  Constant : Constant  Value=0
  Constant1 : Constant  Value=0
  Enabled Subsystem : Subsystem  TreatAsAtomicUnit=on
  LessThanOrEqual : RelationalOperator  OutDataTypeStr=boolean  RndMeth=Simplest  InputSameDT=off
  LessThanOrEqual1 : RelationalOperator  OutDataTypeStr=boolean  RndMeth=Simplest  InputSameDT=off
  Product : Product
  Out1 : Outport
  wires:
  vmax/1 -> LessThanOrEqual/2
  LessThanOrEqual/1 -> AND/1
  dd/1 -> LessThanOrEqual/1, Product/1
  ddd/1 -> Product/2
  Product/1 -> LessThanOrEqual1/1
  Constant/1 -> LessThanOrEqual1/2
  LessThanOrEqual1/1 -> AND/2
  Constant1/1 -> Enabled Subsystem/1(In1)
  Enabled Subsystem/1(Out1) -> Out1/1
  AND/1 -> Enabled Subsystem/Enable

== system massbalancer/Subsystem1/Subsystem1/Subsystem2 ==
  ddd : Inport
  Abs : Abs  SaturateOnIntegerOverflow=off
  Constant1 : Constant  Value=0
  Enabled Subsystem : Subsystem  TreatAsAtomicUnit=on
  LessThanOrEqual : RelationalOperator  OutDataTypeStr=boolean  RndMeth=Simplest  InputSameDT=off
  Out1 : Outport
  wires:
  Abs/1 -> LessThanOrEqual/1
  ddd/1 -> Abs/1
  [Amax] -> LessThanOrEqual/2
  Enabled Subsystem/1(Out1) -> Out1/1
  Constant1/1 -> Enabled Subsystem/1(In1)
  LessThanOrEqual/1 -> Enabled Subsystem/Enable

== system massbalancer/Subsystem1/Subsystem2/Subsystem ==
  d : Inport
  ddd : Inport  Port=2
  dmax : Inport  Port=3
  AND : Logic  IconShape=distinctive  AllPortsSameDT=off  OutDataTypeStr=boolean
  Abs : Abs  SaturateOnIntegerOverflow=off
  Constant : Constant  Value=0  VectorParams1D=off
  Constant1 : Constant  Value=0  VectorParams1D=off
  Enabled Subsystem : Subsystem  TreatAsAtomicUnit=on
  LessThanOrEqual : RelationalOperator  OutDataTypeStr=boolean  RndMeth=Simplest  InputSameDT=off
  LessThanOrEqual1 : RelationalOperator  OutDataTypeStr=boolean  RndMeth=Simplest  InputSameDT=off
  Product : Product
  Out1 : Outport
  wires:
  LessThanOrEqual/1 -> AND/1
  dmax/1 -> LessThanOrEqual/2
  ddd/1 -> Product/2
  Product/1 -> LessThanOrEqual1/1
  Constant/1 -> LessThanOrEqual1/2
  LessThanOrEqual1/1 -> AND/2
  Constant1/1 -> Enabled Subsystem/1(In1)
  Enabled Subsystem/1(Out1) -> Out1/1
  d/1 -> Product/1, Abs/1
  Abs/1 -> LessThanOrEqual/1
  AND/1 -> Enabled Subsystem/Enable

== system massbalancer/Subsystem1/Subsystem2/Subsystem1 ==
  ddd : Inport
  dd : Inport  Port=2
  vmax : Inport  Port=3
  AND : Logic  IconShape=distinctive  AllPortsSameDT=off  OutDataTypeStr=boolean
  Constant : Constant  Value=0
  Constant1 : Constant  Value=0
  Enabled Subsystem : Subsystem  TreatAsAtomicUnit=on
  LessThanOrEqual : RelationalOperator  OutDataTypeStr=boolean  RndMeth=Simplest  InputSameDT=off
  LessThanOrEqual1 : RelationalOperator  OutDataTypeStr=boolean  RndMeth=Simplest  InputSameDT=off
  Product : Product
  Out1 : Outport
  wires:
  Constant1/1 -> Enabled Subsystem/1(In1)
  LessThanOrEqual1/1 -> AND/2
  Constant/1 -> LessThanOrEqual1/2
  Product/1 -> LessThanOrEqual1/1
  ddd/1 -> Product/2
  dd/1 -> Product/1, LessThanOrEqual/1
  LessThanOrEqual/1 -> AND/1
  vmax/1 -> LessThanOrEqual/2
  Enabled Subsystem/1(Out1) -> Out1/1
  AND/1 -> Enabled Subsystem/Enable

== system massbalancer/Subsystem1/Subsystem2/Subsystem2 ==
  ddd : Inport
  Abs : Abs  SaturateOnIntegerOverflow=off
  Constant1 : Constant  Value=0
  Enabled Subsystem : Subsystem  TreatAsAtomicUnit=on
  LessThanOrEqual : RelationalOperator  OutDataTypeStr=boolean  RndMeth=Simplest  InputSameDT=off
  Out1 : Outport
  wires:
  Constant1/1 -> Enabled Subsystem/1(In1)
  Enabled Subsystem/1(Out1) -> Out1/1
  [Amax] -> LessThanOrEqual/2
  ddd/1 -> Abs/1
  Abs/1 -> LessThanOrEqual/1
  LessThanOrEqual/1 -> Enabled Subsystem/Enable

== system massbalancer/Subsystem1/Subsystem3/Subsystem ==
  d : Inport
  ddd : Inport  Port=2
  dmax : Inport  Port=3
  AND : Logic  IconShape=distinctive  AllPortsSameDT=off  OutDataTypeStr=boolean
  Abs : Abs  SaturateOnIntegerOverflow=off
  Constant : Constant  Value=0  VectorParams1D=off
  Constant1 : Constant  Value=0  VectorParams1D=off
  Enabled Subsystem : Subsystem  TreatAsAtomicUnit=on
  LessThanOrEqual : RelationalOperator  OutDataTypeStr=boolean  RndMeth=Simplest  InputSameDT=off
  LessThanOrEqual1 : RelationalOperator  OutDataTypeStr=boolean  RndMeth=Simplest  InputSameDT=off
  Product : Product
  Out1 : Outport
  wires:
  LessThanOrEqual/1 -> AND/1
  dmax/1 -> LessThanOrEqual/2
  ddd/1 -> Product/2
  Product/1 -> LessThanOrEqual1/1
  Constant/1 -> LessThanOrEqual1/2
  LessThanOrEqual1/1 -> AND/2
  Constant1/1 -> Enabled Subsystem/1(In1)
  Enabled Subsystem/1(Out1) -> Out1/1
  d/1 -> Product/1, Abs/1
  Abs/1 -> LessThanOrEqual/1
  AND/1 -> Enabled Subsystem/Enable

== system massbalancer/Subsystem1/Subsystem3/Subsystem1 ==
  ddd : Inport
  dd : Inport  Port=2
  vmax : Inport  Port=3
  AND : Logic  IconShape=distinctive  AllPortsSameDT=off  OutDataTypeStr=boolean
  Constant : Constant  Value=0
  Constant1 : Constant  Value=0
  Enabled Subsystem : Subsystem  TreatAsAtomicUnit=on
  LessThanOrEqual : RelationalOperator  OutDataTypeStr=boolean  RndMeth=Simplest  InputSameDT=off
  LessThanOrEqual1 : RelationalOperator  OutDataTypeStr=boolean  RndMeth=Simplest  InputSameDT=off
  Product : Product
  Out1 : Outport
  wires:
  Enabled Subsystem/1(Out1) -> Out1/1
  Constant1/1 -> Enabled Subsystem/1(In1)
  AND/1 -> Enabled Subsystem/Enable
  LessThanOrEqual1/1 -> AND/2
  Constant/1 -> LessThanOrEqual1/2
  Product/1 -> LessThanOrEqual1/1
  ddd/1 -> Product/2
  dd/1 -> Product/1, LessThanOrEqual/1
  LessThanOrEqual/1 -> AND/1
  vmax/1 -> LessThanOrEqual/2

== system massbalancer/Subsystem1/Subsystem3/Subsystem2 ==
  ddd : Inport
  Abs : Abs  SaturateOnIntegerOverflow=off
  Constant1 : Constant  Value=0
  Enabled Subsystem : Subsystem  TreatAsAtomicUnit=on
  LessThanOrEqual : RelationalOperator  OutDataTypeStr=boolean  RndMeth=Simplest  InputSameDT=off
  Out1 : Outport
  wires:
  Constant1/1 -> Enabled Subsystem/1(In1)
  Enabled Subsystem/1(Out1) -> Out1/1
  [Amax] -> LessThanOrEqual/2
  ddd/1 -> Abs/1
  Abs/1 -> LessThanOrEqual/1
  LessThanOrEqual/1 -> Enabled Subsystem/Enable

== system massbalancer/TNet/Subsystem1/R_I ==
  In1 : Inport
  Add : Sum
  Displacment D : Constant  Value=[0.05;-0.03;0.02]  VectorParams1D=off
  Matrix Concatenate1 : Concatenate  NumInputs=3  Mode=Multidimensional array  ConcatenateDimension=2
  Product : Product
  Product1 : Product
  Product2 : Product
  Selector : Selector  InputPortWidth=3  IndexOptions=Index vector (dialog)  Indices=[1]  OutputSizes=1
  Selector1 : Selector  InputPortWidth=3  IndexOptions=Index vector (dialog)  Indices=[2]  OutputSizes=1
  Selector2 : Selector  InputPortWidth=3  IndexOptions=Index vector (dialog)  Indices=[3]  OutputSizes=1
  Subsystem3 : Subsystem
  Subsystem4 : Subsystem
  Sum1 : Sum  Inputs=|++
  Sum2 : Sum  Inputs=|++
  R_0 : Outport
  wires:
  Subsystem4/1(Out1) -> Add/1
  Product1/1 -> Sum1/1
  Selector1/1 -> Product1/1
  Selector/1 -> Product/1
  Subsystem3/2(Out2) -> Product1/2
  Selector2/1 -> Product2/1
  Subsystem4/2(Out2) -> Sum1/2
  Displacment D/1 -> Selector/1, Selector1/1, Selector2/1
  Subsystem4/3(Out3) -> Sum2/2
  Product/1 -> Add/2
  Subsystem3/1(Out1) -> Product/2
  [s] -> Subsystem3/1(In1)
  Subsystem3/3(Out3) -> Product2/2
  Product2/1 -> Sum2/1
  In1/1 -> Subsystem4/1(In1)
  Add/1 -> Matrix Concatenate1/1
  Sum1/1 -> Matrix Concatenate1/2
  Sum2/1 -> Matrix Concatenate1/3
  Matrix Concatenate1/1 -> R_0/1

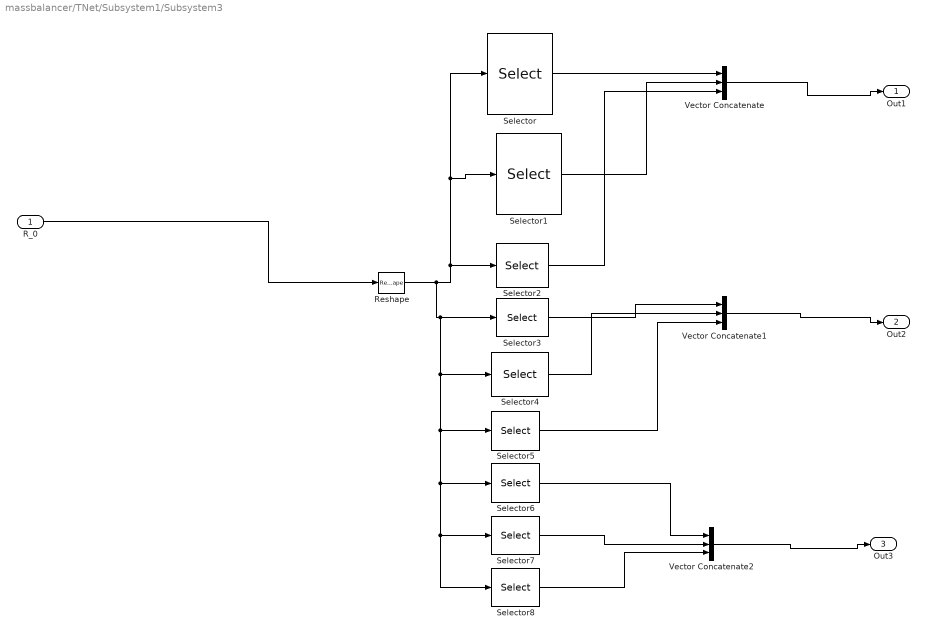
== system massbalancer/TNet/Subsystem1/Subsystem3 ==
  R_0 : Inport
  Reshape : Reshape  OutputDimensionality=Column vector (2-D)  OutputDimensions=[1,3]
  Selector : Selector  InputPortWidth=9  IndexOptions=Index vector (dialog)  Indices=[1]  OutputSizes=1
  Selector1 : Selector  InputPortWidth=9  IndexOptions=Index vector (dialog)  Indices=[2]  OutputSizes=1
  Selector2 : Selector  InputPortWidth=9  IndexOptions=Index vector (dialog)  Indices=[3]  OutputSizes=1
  Selector3 : Selector  InputPortWidth=9  IndexOptions=Index vector (dialog)  Indices=[4]  OutputSizes=1
  Selector4 : Selector  InputPortWidth=9  IndexOptions=Index vector (dialog)  Indices=[5]  OutputSizes=1
  Selector5 : Selector  InputPortWidth=9  IndexOptions=Index vector (dialog)  Indices=[6]  OutputSizes=1
  Selector6 : Selector  InputPortWidth=9  IndexOptions=Index vector (dialog)  Indices=[7]  OutputSizes=1
  Selector7 : Selector  InputPortWidth=9  IndexOptions=Index vector (dialog)  Indices=[8]  OutputSizes=1
  Selector8 : Selector  InputPortWidth=9  IndexOptions=Index vector (dialog)  Indices=[9]  OutputSizes=1
  Vector Concatenate : Concatenate  NumInputs=3  Mode=Multidimensional array
  Vector Concatenate1 : Concatenate  NumInputs=3  Mode=Multidimensional array
  Vector Concatenate2 : Concatenate  NumInputs=3  Mode=Multidimensional array
  Out1 : Outport
  Out2 : Outport  Port=2
  Out3 : Outport  Port=3
  wires:
  Selector2/1 -> Vector Concatenate/3
  Vector Concatenate/1 -> Out1/1
  Selector8/1 -> Vector Concatenate2/3
  Selector4/1 -> Vector Concatenate1/2
  Selector6/1 -> Vector Concatenate2/1
  R_0/1 -> Reshape/1
  Reshape/1 -> Selector8/1, Selector7/1, Selector6/1, Selector5/1, Selector4/1, Selector3/1, Selector2/1, Selector1/1, Selector/1
  Selector/1 -> Vector Concatenate/1
  Selector5/1 -> Vector Concatenate1/3
  Selector7/1 -> Vector Concatenate2/2
  Vector Concatenate2/1 -> Out3/1
  Vector Concatenate1/1 -> Out2/1
  Selector1/1 -> Vector Concatenate/2
  Selector3/1 -> Vector Concatenate1/1

== system massbalancer/TNet/Subsystem1/Tbalances Init T Gravity  ==
  Cross Product : matrix_library/Cross Product
  Display : Display
  Fgravity : Subsystem
  Subsystem : Subsystem
  Out1 : Outport
  Out2 : Outport  Port=2
  wires:
  Subsystem/1(Output) -> Cross Product/1
  Fgravity/1(Out1) -> Out2/1, Cross Product/2
  Cross Product/1 -> Display/1, Out1/1

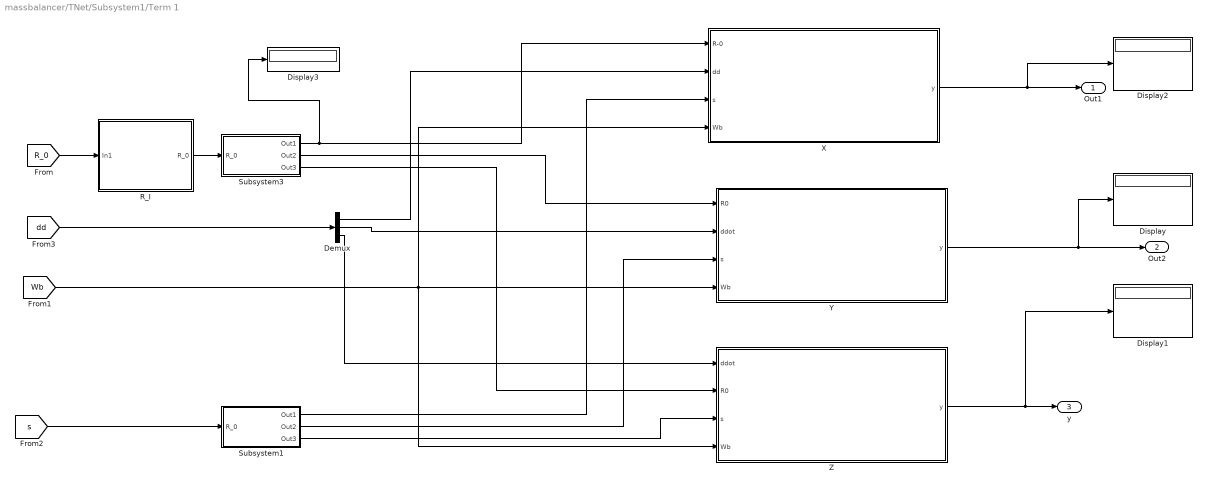
== system massbalancer/TNet/Subsystem1/Term 1 ==
  Demux : Demux  Outputs=3
  Display{,1..3} (4 alike) : Display
  R_I : Subsystem
  Subsystem1 : Subsystem
  Subsystem3 : Subsystem
  X : Subsystem
  Y : Subsystem
  Z : Subsystem
  Out1 : Outport
  Out2 : Outport  Port=2
  y : Outport  Port=3
  wires:
  [R_0] -> R_I/1(In1)
  [s] -> Subsystem1/1(R_0)
  Demux/1 -> X/2(dd)
  R_I/1(R_0) -> Subsystem3/1(R_0)
  Subsystem3/1(Out1) -> X/1(R-0), Display3/1
  Subsystem1/2(Out2) -> Y/3(s)
  Subsystem1/1(Out1) -> X/3(s)
  Subsystem1/3(Out3) -> Z/3(s)
  Subsystem3/3(Out3) -> Z/2(R0)
  [dd] -> Demux/1
  Subsystem3/2(Out2) -> Y/1(R0)
  Demux/3 -> Z/1(ddot)
  [Wb] -> X/4(Wb), Z/4(Wb), Y/4(Wb)
  Y/1(y) -> Display/1, Out2/1
  X/1(y) -> Display2/1, Out1/1
  Demux/2 -> Y/2(ddot)
  Z/1(y) -> Display1/1, y/1

== system massbalancer/TNet/Subsystem1/Term2 ==
  Demux : Demux  Outputs=3
  Display : Display
  R_I : Subsystem
  Subsystem1 : Subsystem
  Subsystem3 : Subsystem
  X : Subsystem
  Y : Subsystem
  Z : Subsystem
  Output : Outport
  Output1 : Outport  Port=2
  Output2 : Outport  Port=3
  wires:
  Subsystem1/1(Out1) -> X/3(s)
  Demux/1 -> X/2(Ddot)
  [dd] -> Demux/1
  Subsystem3/1(Out1) -> X/1(R-0)
  Demux/2 -> Y/2(ddot)
  Subsystem3/3(Out3) -> Z/2(R0)
  Subsystem3/2(Out2) -> Y/1(R0)
  [Wb] -> Z/4(Wb), X/4(Wb), Y/4(Wb)
  Demux/3 -> Z/1(ddot)
  [s] -> Subsystem1/1(R_0)
  Subsystem1/2(Out2) -> Y/3(s)
  [R_0] -> R_I/1(In1)
  Subsystem1/3(Out3) -> Z/3(s)
  X/1(Output) -> Output/1
  Y/1(Output) -> Display/1, Output1/1
  Z/1(Output1) -> Output2/1
  R_I/1(R_0) -> Subsystem3/1(R_0)

== system massbalancer/TNet/Subsystem1/Term3 ==
  Demux : Demux  Outputs=3
  Display{,1..3} (4 alike) : Display
  Subsystem1 : Subsystem
  Subsystem3 : Subsystem
  X : Subsystem
  Y : Subsystem
  Z : Subsystem
  Output : Outport
  Output1 : Outport  Port=2
  Output2 : Outport  Port=3
  wires:
  Subsystem3/1(Out1) -> X/3(r)
  Subsystem3/2(Out2) -> Y/3(r)
  Subsystem3/3(Out3) -> Z/1(r)
  Demux/1 -> X/1(ddoubledot)
  Demux/2 -> Y/1(ddoubledot)
  Demux/3 -> Z/3(ddoubledot)
  [s] -> Subsystem1/1(R_0)
  Subsystem1/1(Out1) -> X/2(s)
  Subsystem1/2(Out2) -> Y/2(s)
  Subsystem1/3(Out3) -> Z/2(s)
  X/1(y) -> Display2/1, Output/1
  Y/1(y) -> Display/1, Output1/1
  Z/1(y) -> Display1/1, Output2/1
  [R_0] -> Subsystem3/1(R_0), Display3/1
  [ddd] -> Demux/1

== system massbalancer/TNet/TBalances/R_I ==
  In1 : Inport
  Add : Sum
  Matrix Concatenate1 : Concatenate  NumInputs=3  Mode=Multidimensional array  ConcatenateDimension=2
  Product : Product
  Product1 : Product
  Product2 : Product
  Selector : Selector  InputPortWidth=3  IndexOptions=Index vector (dialog)  Indices=[1]  OutputSizes=1
  Selector1 : Selector  InputPortWidth=3  IndexOptions=Index vector (dialog)  Indices=[2]  OutputSizes=1
  Selector2 : Selector  InputPortWidth=3  IndexOptions=Index vector (dialog)  Indices=[3]  OutputSizes=1
  Subsystem3 : Subsystem
  Subsystem4 : Subsystem
  Sum1 : Sum  Inputs=|++
  Sum2 : Sum  Inputs=|++
  R_0 : Outport
  wires:
  Subsystem4/1(Out1) -> Add/1
  Product1/1 -> Sum1/1
  Selector1/1 -> Product1/1
  Selector/1 -> Product/1
  Subsystem3/2(Out2) -> Product1/2
  Selector2/1 -> Product2/1
  Subsystem4/2(Out2) -> Sum1/2
  In1/1 -> Selector/1, Selector1/1, Selector2/1
  Subsystem4/3(Out3) -> Sum2/2
  Product/1 -> Add/2
  Subsystem3/1(Out1) -> Product/2
  [S] -> Subsystem3/1(In1)
  Subsystem3/3(Out3) -> Product2/2
  Product2/1 -> Sum2/1
  [R_0] -> Subsystem4/1(In1)
  Add/1 -> Matrix Concatenate1/1
  Sum1/1 -> Matrix Concatenate1/2
  Sum2/1 -> Matrix Concatenate1/3
  Matrix Concatenate1/1 -> R_0/1

== system massbalancer/TNet/TBalances/Term1 ==
  dd : Inport
  S : Inport  Port=2
  R_0 : Inport  Port=3
  Wb : Inport  Port=4
  Demux : Demux  Outputs=3
  Subsystem1 : Subsystem
  Subsystem3 : Subsystem
  X : Subsystem
  Y : Subsystem
  Z : Subsystem
  Output : Outport
  Output1 : Outport  Port=2
  Output2 : Outport  Port=3
  wires:
  R_0/1 -> Subsystem3/1(R_0)
  Subsystem3/1(Out1) -> X/1(R-0)
  Subsystem3/2(Out2) -> Y/1(R0)
  Subsystem3/3(Out3) -> Z/2(R0)
  dd/1 -> Demux/1
  Demux/1 -> X/2(dd)
  Demux/2 -> Y/2(ddot)
  Wb/1 -> Z/4(Wb), X/4(Wb), Y/4(Wb)
  Demux/3 -> Z/1(ddot)
  S/1 -> Subsystem1/1(R_0)
  Subsystem1/1(Out1) -> X/3(s)
  Subsystem1/2(Out2) -> Y/3(s)
  Subsystem1/3(Out3) -> Z/3(s)
  X/1(y) -> Output/1
  Y/1(y) -> Output1/1
  Z/1(y) -> Output2/1

== system massbalancer/TNet/TBalances/Term2 ==
  ddot : Inport
  r0 : Inport  Port=2
  s : Inport  Port=3
  wb : Inport  Port=4
  Demux : Demux  Outputs=3
  Display : Display
  Display2 : Display
  Subsystem1 : Subsystem
  Subsystem3 : Subsystem
  X : Subsystem
  Y : Subsystem
  Z : Subsystem
  Output : Outport
  Output1 : Outport  Port=2
  Output2 : Outport  Port=3
  wires:
  Subsystem1/1(Out1) -> X/3(s)
  Demux/1 -> X/2(Ddot)
  ddot/1 -> Demux/1
  Subsystem3/1(Out1) -> X/1(R-0)
  Demux/2 -> Y/2(ddot)
  Subsystem3/3(Out3) -> Z/2(R0)
  Subsystem3/2(Out2) -> Y/1(R0)
  wb/1 -> Z/4(Wb), X/4(Wb), Y/4(Wb)
  Demux/3 -> Z/1(ddot)
  s/1 -> Subsystem1/1(R_0)
  Subsystem1/2(Out2) -> Y/3(s)
  r0/1 -> Subsystem3/1(R_0)
  Subsystem1/3(Out3) -> Z/3(s)
  X/1(Output) -> Display2/1, Output/1
  Y/1(Output) -> Output1/1
  Z/1(Output1) -> Display/1, Output2/1

== system massbalancer/TNet/TBalances/Term3 ==
  r : Inport
  ddoubledot : Inport  Port=2
  s : Inport  Port=3
  Demux : Demux  Outputs=3
  Display : Display
  Display1 : Display
  Display2 : Display
  Subsystem1 : Subsystem
  Subsystem3 : Subsystem
  X : Subsystem
  Y : Subsystem
  Z : Subsystem
  Output : Outport
  Output1 : Outport  Port=2
  Output2 : Outport  Port=3
  wires:
  r/1 -> Subsystem3/1(R_0)
  ddoubledot/1 -> Demux/1
  Subsystem3/1(Out1) -> X/3(r)
  Subsystem3/2(Out2) -> Y/3(r)
  Subsystem3/3(Out3) -> Z/1(r)
  Demux/1 -> X/1(ddoubledot)
  Demux/2 -> Y/1(ddoubledot)
  Demux/3 -> Z/3(ddoubledot)
  s/1 -> Subsystem1/1(R_0)
  Subsystem1/1(Out1) -> X/2(s)
  Subsystem1/2(Out2) -> Y/2(s)
  Subsystem1/3(Out3) -> Z/2(s)
  X/1(y) -> Display2/1, Output/1
  Y/1(y) -> Display/1, Output1/1
  Z/1(y) -> Display1/1, Output2/1

== system massbalancer/TNet/Tbalances Init T Gravity /Fgravity ==
  Matrix Multiply : Product  Multiplication=Matrix(*)
  Q(q) rotational form of quaternio : Subsystem
  Out1 : Outport
  wires:
  Q(q) rotational form of quaternio/1(Out1) -> Matrix Multiply/1
  [G] -> Matrix Multiply/2
  [q] -> Q(q) rotational form of quaternio/1(Q_input)
  Matrix Multiply/1 -> Out1/1

== system massbalancer/TNet/Tbalances Init T Gravity /Subsystem ==
  Subsystem2 : Subsystem
  Output : Outport
  wires:
  [M_r] -> Subsystem2/1(In1)
  Subsystem2/1(Output) -> Output/1

== system massbalancer/Wdot b/I_r/Subsystem ==
  In1 : Inport
  Constant : Constant  Value=0  VectorParams1D=off
  Constant1 : Constant  Value=0  VectorParams1D=off
  Constant2 : Constant  Value=0  VectorParams1D=off
  Demux : Demux  Outputs=3
  Gain : Gain  Gain=-1
  Gain1 : Gain  Gain=-1
  Gain2 : Gain  Gain=-1
  Matrix Concatenate : Concatenate  NumInputs=3  Mode=Multidimensional array  ConcatenateDimension=2
  Mux : Mux  Inputs=3
  Mux1 : Mux  Inputs=3
  Mux2 : Mux  Inputs=3
  Out1 : Outport
  wires:
  Constant/1 -> Mux/1
  Gain2/1 -> Mux2/1
  Gain1/1 -> Mux1/3
  Mux/1 -> Matrix Concatenate/1
  Demux/2 -> Mux/3, Gain2/1
  In1/1 -> Demux/1
  Gain/1 -> Mux/2
  Demux/3 -> Mux1/1, Gain/1
  Mux1/1 -> Matrix Concatenate/2
  Mux2/1 -> Matrix Concatenate/3
  Demux/1 -> Mux2/2, Gain1/1
  Constant1/1 -> Mux1/2
  Constant2/1 -> Mux2/3
  Matrix Concatenate/1 -> Out1/1

== system massbalancer/Wdot b/I_r/Subsystem1 ==
  In1 : Inport
  Constant : Constant  Value=0  VectorParams1D=off
  Constant1 : Constant  Value=0  VectorParams1D=off
  Constant2 : Constant  Value=0  VectorParams1D=off
  Demux : Demux  Outputs=3
  Gain : Gain  Gain=-1
  Gain1 : Gain  Gain=-1
  Gain2 : Gain  Gain=-1
  Matrix Concatenate : Concatenate  NumInputs=3  Mode=Multidimensional array  ConcatenateDimension=2
  Mux : Mux  Inputs=3
  Mux1 : Mux  Inputs=3
  Mux2 : Mux  Inputs=3
  Out1 : Outport
  wires:
  Matrix Concatenate/1 -> Out1/1
  Constant2/1 -> Mux2/3
  Constant1/1 -> Mux1/2
  Demux/1 -> Gain1/1, Mux2/2
  Mux2/1 -> Matrix Concatenate/3
  Mux1/1 -> Matrix Concatenate/2
  Demux/3 -> Gain/1, Mux1/1
  Gain/1 -> Mux/2
  In1/1 -> Demux/1
  Demux/2 -> Gain2/1, Mux/3
  Mux/1 -> Matrix Concatenate/1
  Gain1/1 -> Mux1/3
  Gain2/1 -> Mux2/1
  Constant/1 -> Mux/1

== system massbalancer/Wdot b/I_r/Subsystem2 ==
  In1 : Inport
  Constant : Constant  Value=0  VectorParams1D=off
  Constant1 : Constant  Value=0  VectorParams1D=off
  Constant2 : Constant  Value=0  VectorParams1D=off
  Demux : Demux  Outputs=3
  Gain : Gain  Gain=-1
  Gain1 : Gain  Gain=-1
  Gain2 : Gain  Gain=-1
  Matrix Concatenate : Concatenate  NumInputs=3  Mode=Multidimensional array  ConcatenateDimension=2
  Mux : Mux  Inputs=3
  Mux1 : Mux  Inputs=3
  Mux2 : Mux  Inputs=3
  Out1 : Outport
  wires:
  Constant/1 -> Mux/1
  Gain2/1 -> Mux2/1
  Gain1/1 -> Mux1/3
  Mux/1 -> Matrix Concatenate/1
  Demux/2 -> Mux/3, Gain2/1
  In1/1 -> Demux/1
  Gain/1 -> Mux/2
  Demux/3 -> Mux1/1, Gain/1
  Mux1/1 -> Matrix Concatenate/2
  Mux2/1 -> Matrix Concatenate/3
  Demux/1 -> Mux2/2, Gain1/1
  Constant1/1 -> Mux1/2
  Constant2/1 -> Mux2/3
  Matrix Concatenate/1 -> Out1/1
